simulink model "Parsim_for_3level"  (R2024b)
settings: Solver=FixedStepDiscrete  StartTime=0.0  StopTime=1  FixedStep=Ts  RelTol=1e-3
PreLoadFcn:
  | Net_improve_init;L=Lac_MV;Ts=20e-6;Tctrl=Ts;Rac_MV=1;
PostLoadFcn:
  | Net_improve_init;L=Lac_MV;Ts=20e-6;Tctrl=Ts;Rac_MV=1;
InitFcn:
  | Net_improve_init;L=Lac_MV;Ts=20e-6;Tctrl=Ts;Rac_MV=1;
undefined symbols (not defined in the file or in its folder): C1, dend, DiscIntNeverNeededParam, fs, Lac_MV, numd, Pref, R1, Vac_peak_MV, Vdc
libraries: spsIGBTDiodeLib x12, powerlib_extras x10, spsControlledVoltageSourceLib x8, spsCurrentMeasurementLib x6, spsSeriesRLCBranchLib x6, spsVoltageMeasurementLib x6, spsThreePhaseVIMeasurementLib x4, spsGroundLib x4, spsIdealSwitchLib x2, spsPower3phInstantaneousLib x2, simulink x2, spsThreePhaseSeriesRLCBranchLib x2
(part 1 of 2)
Description:
  | The Model initialization function Callback automatically
  | 
  | sets the sample time  to 2e-6 sec.  and loads the initial
  | 
  | states vector xInitial. The initial state vector is saved in the
  | 
  | power_acdrive_init.mat file.
  | 
  | 
  | 
  | Check  the Initial state checkbox in the Simulation
  | 
  | parameters/Workspace I/O to start in steady state with a
  | 
  | speed of 120 rad/s and a torque of 0 N.m/s,
  | 
  | 
  | Copyright 2008-2015 The MathWorks, Inc.
settings Model: Creator=WeiLi  LastModifiedBy=KeXing
settings SolverCC: AlgebraicLoopSolver=TrustRegion
settings DataIOCC: SaveFinalState=on  SaveFormat=Array  SignalLoggingSaveFormat=ModelDataLogs  SaveOutput=off  SaveTime=off  ReturnWorkspaceOutputs=off  SignalLoggingName=sigsOut
settings OptimizationCC: BlockReduction=off  ExpressionDepthLimit=2147483647  InitFltsAndDblsToZero=on  LifeSpan=inf
settings DebuggingCC: SaveWithParameterizedLinksMsg=none  UnderspecifiedInitializationDetection=Classic  MergeDetectMultiDrivingBlocksExec=none  CheckExecutionContextPreStartOutputMsg=on  SignalResolutionControl=TryResolveAllWithWarning  MultiTaskDSMMsg=warning  MultiTaskCondExecSysMsg=none  FcnCallInpInsideContextMsg=warning  UnconnectedInputMsg=warning  UnconnectedLineMsg=warning  StateNameClashWarn=warning  SFUnexpectedBacktrackingDiag=warning  SFNoUnconditionalDefaultTransitionDiag=warning  SFExecutionAtInitializationDiag=none  ArithmeticOperatorsInVariantConditions=warning
settings HardwareCC: ProdBitPerPointer=32  ProdBitPerSizeT=32  ProdBitPerPtrDiffT=32  ProdLargestAtomicFloat=None  ProdIntDivRoundTo=Undefined  ProdEndianess=Unspecified  ProdWordSize=32  ProdHWDeviceType=32-bit Generic  TargetUnknown=on
settings ModelReferenceCC: EnableRefExpFcnMdlSchedulingChecks=on  PropagateSignalLabelsOutOfModel=off
settings SFSimCC: SimUseLocalCustomCode=off  CustomCodeUndefinedFunction=UseInterfaceOnly
settings RTWCC: RTWUseLocalCustomCode=off  GPUComputeCapability=3.5
settings CodeAppCC: StateflowObjectComments=on
settings GRTTargetCC: TargetFcnLib=ansi_tfl_tmw.mat  TargetLangStandard=C89/C90 (ANSI)  CombineOutputUpdateFcns=off  GRTInterface=on
settings ConfigComp: CovMetricSettings=dw  CovSaveCumulativeToWorkspaceVar=on  CovSaveSingleToWorkspaceVar=on  CovExternalEMLEnable=off
settings SimscapeCC: SimscapeNormalizeSystem=off

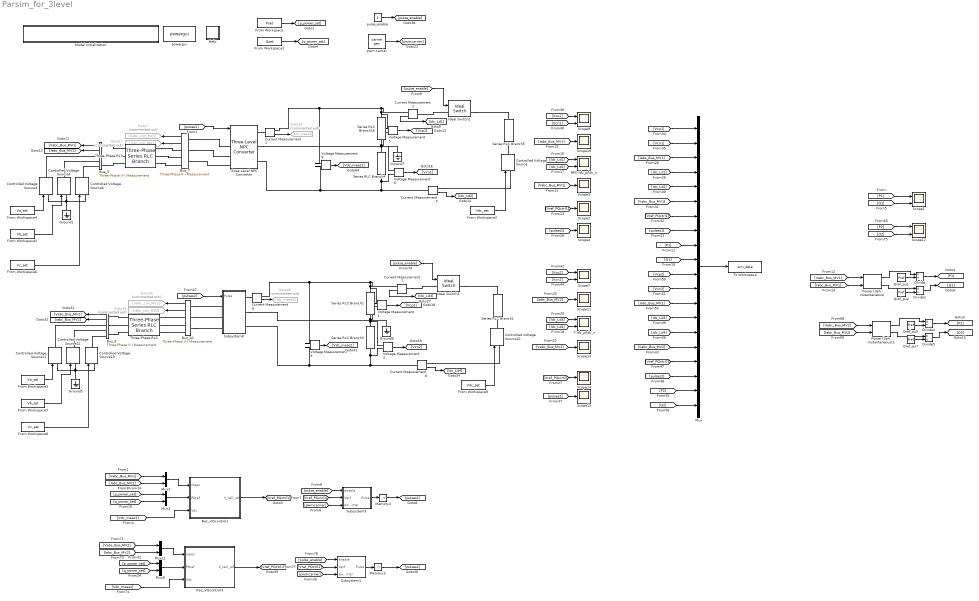
== system Parsim_for_3level ==
  Bus_{5,7,9..10} (4 alike) : spsThreePhaseVIMeasurementLib/Three-Phase V-I Measurement  VoltageMeasurement=phase-to-ground  SetLabelV=off  LabelV=Vabc  Vpu=off  VpuLL=off  CurrentMeasurement=yes  SetLabelI=off  LabelI=Iabc  Ipu=off  Pbase=P_AC  Vbase=V_AC_prim  OutputType=Complex  PhasorSimulation=off  PSBequivalent=0
  Controlled Voltage Source : spsControlledVoltageSourceLib/Controlled Voltage Source  Initialize=on  Source_Type=DC  Amplitude=3000  Phase=0  Frequency=0  Measurements=None
  Controlled Voltage Source10 : spsControlledVoltageSourceLib/Controlled Voltage Source  Initialize=on  Source_Type=DC  Amplitude=3000  Phase=0  Frequency=0  Measurements=None
  Controlled Voltage Source{3..4,6,11..13} (6 alike) : spsControlledVoltageSourceLib/Controlled Voltage Source  Initialize=off  Source_Type=AC  Amplitude=0  Phase=0  Frequency=fs  Measurements=None
  Current Measurement{1..2,5..8} (6 alike) : spsCurrentMeasurementLib/Current Measurement  PhasorSimulation=off  OutputType=Complex  PSBequivalent=0
  Divide{,1,4..5} (4 alike) : Product  Inputs=*/
  From Workspace : FromWorkspace  VariableName=Pset
  From Workspace1 : FromWorkspace  VariableName=Qset
  From Workspace2 : FromWorkspace  VariableName=Vdc_set  SampleTime=Ts
  From Workspace3 : FromWorkspace  VariableName=Va_set  SampleTime=Ts
  From Workspace4 : FromWorkspace  VariableName=Va_set  SampleTime=Ts
  From Workspace5 : FromWorkspace  VariableName=Vb_set  SampleTime=Ts
  From Workspace6 : FromWorkspace  VariableName=Vc_set  SampleTime=Ts
  From Workspace7 : FromWorkspace  VariableName=Vb_set  SampleTime=Ts
  From Workspace8 : FromWorkspace  VariableName=Vc_set  SampleTime=Ts
  From Workspace9 : FromWorkspace  VariableName=Vdc_set  SampleTime=Ts
  Goto10 : Goto  Commented=on  GotoTag=Idc_meas1
  Goto17 : Goto  Commented=on  GotoTag=iabc_con_MV1
  Goto28 : Goto  Commented=on  GotoTag=Idc_meas2
  Goto30 : Goto  Commented=on  GotoTag=Vabc_con_MV2
  Goto33 : Goto  Commented=on  GotoTag=iabc_con_MV2
  Goto7 : Goto  Commented=on  GotoTag=Vabc_con_MV1
  Ground{1,5..7} (4 alike) : spsGroundLib/Ground  LConnTagsString=a
  Help : Subsystem  mask(OpDoc){docfile=../Help/help.html}
      mask init:
      | %patch([1,1,0,0,.8,1],[.8,0,0,1,1,.8],[.8 .8 .8]);
      | %patch([.15 .78 .78 .15 .15],[.8 .8 .83 .83 .8],[.9 .9 .9]);
      | %patch([.15 .78 .78 .15 .15],[.7 .7 .73 .73 .8],[.9 .9 .9]);
      | %patch([.15 .78 .78 .15 .15],[.6 .6 .63 .63 .6],[.9 .9 .9]);
      | %patch([.15 .78 .78 .15 .15],[.5 .5 .53 .53 .5],[.9 .9 .9]);
      | %patch([.15 .78 .78 .15 .15],[.4 .4 .43 .43 .4],[.9 .9 .9]);
      settings: OpenFcn=OpHelp_cb(gcb);
      mask Display: image(imread('opdoc.bmp'))
  Ideal Switch2 : spsIdealSwitchLib/Ideal Switch  Ron=0.001  Lon=0  IC=0  Rs=1e9  Cs=inf  Measurements=on
  Ideal Switch3 : spsIdealSwitchLib/Ideal Switch  Ron=0.001  Lon=0  IC=0  Rs=1e9  Cs=inf  Measurements=on
  Memory2 : Memory
  Memory3 : Memory
  Model Initialization : Subsystem  mask(Model Functions){InitFcnX=Net_improve_init;L=Lac_MV;Ts=20e-6;Tctrl=Ts;Rac_MV=1;, prel=on, posl=on, inif=on, strf=off}
      mask prompts: InitFcnX "Initialisation"; prel "Preload Function"; posl "PostLoad Function"; inif "InitFcn"; strf "StartFcn"
      mask init:
      | currentBlock = gcb;
      | root = bdroot(currentBlock);
      | 
      | if ~strcmp(get_param(root,'BlockDiagramType'),'library')
      |     if prel==1
      |         set_param(root, 'PreLoadFcn', InitFcnX);
      |     else
      |         set_param(root, 'PreLoadFcn', '');
      |     end
      |     if inif==1
      |         set_param(root, 'InitFcn', InitFcnX);
      |     else
      |         set_param(root, 'InitFcn', '');
      |     end
      |     if strf==1
      |         set_param(root, 'StartFcn', InitFcnX);
      |     else
      |         set_param(root, 'StartFcn', '');
      |     end
      |     if posl==1
      |         set_param(root, 'PostLoadFcn', InitFcnX);
      |     else
      |         set_param(root, 'PostLoadFcn', '');
      |     end
      | end
      | 
      | pos = get_param(currentBlock, 'Position');
      | width = pos(3) - pos(1); height = pos(4) - pos(2);
      | txt = [ upper(root) '\n' '- InitFcn. . . . . '  get_param(root, 'InitFcn') ];
      settings: CopyFcn=set_param(gcb,'LinkStatus','none')
      mask Display: text(5, height*0.5, txt, 'horizontalAlignment', 'left', 'verticalAlignment', 'middle') ;
  Mux : Mux  Inputs=20
  Mux{1..2,8,11} (4 alike) : Mux  Inputs=2
  NPC-Idc_p/Idc_n : Scope  NumInputPorts=2
  "Power (3ph, Instantaneous)" : spsPower3phInstantaneousLib/Power (3ph, Instantaneous)
  "Power (3ph, Instantaneous)2" : spsPower3phInstantaneousLib/Power (3ph, Instantaneous)
  Qref_pu{1..2,5,7} (4 alike) : Constant  Value=Pref
  Rec_VQcontrol1 : Subsystem  mask(converter controller){cm=off, base=[Pref, Vac_peak_MV*sqrt(3/2), Vdc/2, fs], LRx=[Lac_MV, Rac_MV], LRx_inpu=off, Kd=[0.3  2]*10/6  %was [1 0.1]   ; [0.1  1]*1, Kp=[0.3 1]*1     %was [1 0.1]   ; [0.1  1]*1, Kvdc=[2 10]*1;   %was [0.5 1]*20 for Cdc=320uF, Vabc_lim=[-1 1], limitVdq=1.1, nadv=6, xtrIctrl1=[0.4 10 10 -10], Ts=Tctrl}
      mask prompts: cm "control mode (check VQ/uncheck PQ), only one terminal in VQ mode"; base "base value for power(VA), ac voltage(V), dc voltage to ground(V), and frequenvy(Hz) [Sb, Vb, Vdcb,freq]"; LRx "commutation inductance and resistance [Lx, Rx]"; LRx_inpu "[Lx, Rx] in pu if checked/ SI unchecked"; Kd "Kp Ki for d-axis PI control [kp ki]"; Kp "Kp Ki for q-axis PI control [kp ki]"; Kvdc "Kp Ki for Vdc PI control [kp ki]"; Vabc_lim "output Vabc limit [min max]"; limitVdq "limit for Vd,Vq (pu, default = 1.1)"; nadv "nb of time step to compesate for delay (default=1)"; xtrIctrl1 "[kp, kp, limitmax, limitmin] for current control (default=[0.4, 10, 10, -10])"
      mask help:
      | input 1, 6 dimentions, Vabc, Iabc, (SI)
      | input 2, 2 dimentions, Pref, Qref (PU)
      | input 3, 6 dimentions, Vcap at up arm a, lower arm a, up arm b, lower arm b, up arm c and lower arm c.
      | input 4, 1 dimention, pulse on
      | input 5, 1 dimention
      |
      | power or current directions: to go into grid is positive
      mask init:
      | if cm==0;
      |     x=['PQ\nmode'];
      | else
      |     x=['VQ\nmode'];
      | end
      | 
      | Sb=base(1);            %VA 3phase power base;
      | Vb=base(2);       %V, line-line rms voltage base
      | Ib=Sb/(sqrt(3)*Vb); %A, rms current base
      | Zb=Vb^2/Sb ;        %ohm, impedence base
      | Vdc=base(3);      %V Vdc+ to ground or ground to Vdc- 
      | frq=base(4);
      | 
      | if LRx_inpu
      |     Rxpu=LRx(2);
      |     Lxpu=LRx(1);
      | else
      |     Rxpu=LRx(2)/Zb;
      |     Lxpu=LRx(1)*2*pi*frq/Zb;
      | end;
      | 
      | ks=Vdc*sqrt(3/2)/Vb;     % ma=1/ks for 1pu dc ->1pu ac;
      | 
      | Kp=Kd;
      mask DialogControl ParameterTabVar0 Prompt: parameters
      mask DialogControl ParameterTabVar01 Prompt: advanced
      mask Display: disp (x);
  Rec_VQcontrol3 : Subsystem  mask(converter controller){cm=off, base=[Pref, Vac_peak_MV*sqrt(3/2), Vdc/2, fs], LRx=[Lac_MV, Rac_MV], LRx_inpu=off, Kd=[0.3  2]*10/6  %was [1 0.1]   ; [0.1  1]*1, Kp=[0.3 1]*1     %was [1 0.1]   ; [0.1  1]*1, Kvdc=[2 10]*1;   %was [0.5 1]*20 for Cdc=320uF, Vabc_lim=[-1 1], limitVdq=1.1, nadv=6, xtrIctrl1=[0.4 10 10 -10], Ts=Tctrl}
      mask prompts: cm "control mode (check VQ/uncheck PQ), only one terminal in VQ mode"; base "base value for power(VA), ac voltage(V), dc voltage to ground(V), and frequenvy(Hz) [Sb, Vb, Vdcb,freq]"; LRx "commutation inductance and resistance [Lx, Rx]"; LRx_inpu "[Lx, Rx] in pu if checked/ SI unchecked"; Kd "Kp Ki for d-axis PI control [kp ki]"; Kp "Kp Ki for q-axis PI control [kp ki]"; Kvdc "Kp Ki for Vdc PI control [kp ki]"; Vabc_lim "output Vabc limit [min max]"; limitVdq "limit for Vd,Vq (pu, default = 1.1)"; nadv "nb of time step to compesate for delay (default=1)"; xtrIctrl1 "[kp, kp, limitmax, limitmin] for current control (default=[0.4, 10, 10, -10])"
      mask help:
      | input 1, 6 dimentions, Vabc, Iabc, (SI)
      | input 2, 2 dimentions, Pref, Qref (PU)
      | input 3, 6 dimentions, Vcap at up arm a, lower arm a, up arm b, lower arm b, up arm c and lower arm c.
      | input 4, 1 dimention, pulse on
      | input 5, 1 dimention
      |
      | power or current directions: to go into grid is positive
      mask init: same as Parsim_for_3level/Rec_VQcontrol1
      mask DialogControl ParameterTabVar0 Prompt: parameters
      mask DialogControl ParameterTabVar01 Prompt: advanced
      mask Display: disp (x);
  Scope{1,7,9,12} (4 alike) : Scope  NumInputPorts=2
  Scope{2..4,10..11,13..15} (8 alike) : Scope
  Series RLC Branch1 : spsSeriesRLCBranchLib/Series RLC Branch  LConnTagsString=__new0  RConnTagsString=__new0  BranchType=R  Resistance=3e3^2/(Pref)/10*2  Inductance=1e-3  SetiL0=off  InitialCurrent=0  Capacitance=C1  Setx0=off  InitialVoltage=0  Measurements=None
  Series RLC Branch{2..4,16} (4 alike) : spsSeriesRLCBranchLib/Series RLC Branch  LConnTagsString=__new0  RConnTagsString=__new0  BranchType=C  Resistance=R1  Inductance=1e-3  SetiL0=off  InitialCurrent=0  Capacitance=C1  Setx0=off  InitialVoltage=0  Measurements=None
  Series RLC Branch5 : spsSeriesRLCBranchLib/Series RLC Branch  LConnTagsString=__new0  RConnTagsString=__new0  BranchType=R  Resistance=3e3^2/(Pref)/10*2  Inductance=1e-3  SetiL0=off  InitialCurrent=0  Capacitance=C1  Setx0=off  InitialVoltage=0  Measurements=None
  Subsystem1 : Subsystem
  Subsystem8 : Subsystem
  Subsystem9 : Subsystem
  T-Idc_p/Idc_n : Scope  NumInputPorts=2
  Three-Level NPC Converter : spsThreeLevelNPCConverterLib/Three-Level NPC Converter  ModelType=Switching devices  Ron=IGBT_Ron  Rs=1e5  Cs=IGBT_Cs  Vforward=[0,0]  Ron_Diode=1e-3  Rs_Diode=1e6  Cs_Diode=inf  Vf_Diode=1e-3  Rs_CurrentSource=inf  Ron_ACsource=1e-3
      settings: LibrarySourceBlock=|
      | sps_lib/Power Electronics/Three-Level
      | NPC Converter
  Three-Phase RL3 : spsThreePhaseSeriesRLCBranchLib/Three-Phase Series RLC Branch  LConnTagsString=A|B|C  RConnTagsString=A|B|C  BranchType=RL  Resistance=Rac_MV  Inductance=Lac_MV  Capacitance=1e-6  Measurements=None
  Three-Phase RL5 : spsThreePhaseSeriesRLCBranchLib/Three-Phase Series RLC Branch  LConnTagsString=A|B|C  RConnTagsString=A|B|C  BranchType=RL  Resistance=Rac_MV  Inductance=Lac_MV  Capacitance=1e-6  Measurements=None
  To Workspace : ToWorkspace  VariableName=sim_data  SampleTime=-1
      settings: Save2DSignal=2-D array (concatenate along first dimension)
  Voltage Measurement{1..3,5..6,8} (6 alike) : spsVoltageMeasurementLib/Voltage Measurement  PhasorSimulation=off  OutputType=Complex  PSBequivalent=0
  powergui : spspowerguiLib/powergui  Priority=2  SimulationMode=Discrete  SampleTime=Ts  frequency=60  Iterations=50  frequencyindice=0  Pbase=100e6  ErrMax=1e-4  UnitsV=kV  UnitsW=MW  buscounter=0  FunctionMessages=off  echomessages=off  EnableUseOfTLC=off  CurrentSourceSwitches=off  DisableSnubberDevices=off  DisableRonSwitches=off  DisableVfSwitches=off  DisplayEquations=off  AutomaticDiscreteSolvers=off  SolverType=Backward Euler  Interpol=off  ExternalGateDelay=off  methode=off  Ts=0  x0status=blocks  SPID=off  SwTol=0  HookPort=off  NonlinearTolerance=1e-4  nMaxIteration=100  ContinueOnMaxIteration=off  RestoreLinks=warning  ResistiveCurrentMeasurement=off  Frange=[0:2:500]  Ylog=off  Xlog=on  ShowGrid=off  save=off  variable=ZData  structure=VI  ZoomFFT=off  StartTime=9  cycles=10  DisplayStyle=2  fundamental=300/pi  FreqAxis=off  MaxFrequency=1000  frequencyindicesteady=1  RmsSteady=1  display=off
  pulse_enable : Constant
  pwm carrier : libMMCcpuv2/carrier gen  fc=f_cari  range=[1 0]  Ms=3  Ns=1
  wires:
  pwm carrier/1 -> [pwmcarrier]
  From Workspace1/1 -> [q_power_set]
  pulse_enable/1 -> [pulse_enable]
  From Workspace/1 -> [p_power_set]
  Current Measurement1/1 -> Goto10/1
  From Workspace2/1 -> Controlled Voltage Source/1
  Bus_5/1 -> [Vabc_Bus_MV1]
  [pulses1] -> Three-Level NPC Converter/1
  Bus_7/1 -> Goto7/1
  Bus_7/2 -> Goto17/1
  [Iabc_Bus_MV1] -> "Power (3ph, Instantaneous)"/2
  [p_power_set] -> Mux1/1
  [Q1] -> Scope1/2
  Mux1/1 -> Rec_VQcontrol1/2(PQref)
  Qref_pu2/1 -> Divide1/2
  Qref_pu1/1 -> Divide/2
  [P1] -> Scope1/1
  [Vdc_meas1] -> Rec_VQcontrol1/3(Vdc)
  Divide1/1 -> [Q1]
  Rec_VQcontrol1/1(V_cell_ref) -> [Vref_PQctrl1]
  [pulse_enable] -> Ideal Switch2/1
  Current Measurement5/1 -> [Idc_Ld2]
  Voltage Measurement6/1 -> [Vcn1]
  Subsystem9/1(Pulse) -> Memory2/1
  [pwmcarrier] -> Subsystem9/3(pwmcarrier)
  Mux2/1 -> Rec_VQcontrol1/1(meas)
  [Vref_PQctrl1] -> Subsystem9/2(Verf)
  [pulse_enable] -> Subsystem9/1(enable)
  Current Measurement2/1 -> [Idc_Ld1]
  [Iabc_Bus_MV1] -> Mux2/2
  Bus_5/2 -> [Iabc_Bus_MV1]
  Voltage Measurement8/1 -> [Vdc_meas1]
  Voltage Measurement5/1 -> [Vcp1]
  From Workspace6/1 -> Controlled Voltage Source6/1
  From Workspace5/1 -> Controlled Voltage Source4/1
  [Vabc_Bus_MV1] -> Mux2/1
  Divide/1 -> [P1]
  Memory2/1 -> [pulses1]
  [Vabc_Bus_MV1] -> "Power (3ph, Instantaneous)"/1
  From Workspace4/1 -> Controlled Voltage Source3/1
  "Power (3ph, Instantaneous)"/1 -> Divide/1
  [q_power_set] -> Mux1/2
  "Power (3ph, Instantaneous)"/2 -> Divide1/1
  [pulse_enable] -> Ideal Switch3/1
  Voltage Measurement3/1 -> [Vdc_meas2]
  From Workspace7/1 -> Controlled Voltage Source12/1
  From Workspace3/1 -> Controlled Voltage Source11/1
  [pwmcarrier] -> Subsystem1/3(pwmcarrier)
  [Vref_PQctrl2] -> Subsystem1/2(Verf)
  Subsystem1/1(Pulse) -> Memory3/1
  [pulse_enable] -> Subsystem1/1(enable)
  Qref_pu5/1 -> Divide4/2
  Memory3/1 -> [pulses2]
  [Iabc_Bus_MV2] -> "Power (3ph, Instantaneous)2"/2
  [Vdc_meas2] -> Rec_VQcontrol3/3(Vdc)
  From Workspace8/1 -> Controlled Voltage Source13/1
  [P2] -> Scope12/1
  Divide5/1 -> [Q2]
  Divide4/1 -> [P2]
  [Q2] -> Scope12/2
  Mux8/1 -> Rec_VQcontrol3/2(PQref)
  "Power (3ph, Instantaneous)2"/1 -> Divide4/1
  Mux11/1 -> Rec_VQcontrol3/1(meas)
  From Workspace9/1 -> Controlled Voltage Source10/1
  Bus_10/2 -> Goto33/1
  Voltage Measurement2/1 -> [Vcn2]
  "Power (3ph, Instantaneous)2"/2 -> Divide5/1
  Bus_9/1 -> [Vabc_Bus_MV2]
  [Vabc_Bus_MV2] -> "Power (3ph, Instantaneous)2"/1
  Current Measurement8/1 -> [Idc_Ld4]
  [Iabc_Bus_MV2] -> Mux11/2
  Current Measurement6/1 -> Goto28/1
  Bus_10/1 -> Goto30/1
  [pulses2] -> Subsystem8/1(Pulse)
  Bus_9/2 -> [Iabc_Bus_MV2]
  [Vabc_Bus_MV2] -> Mux11/1
  Rec_VQcontrol3/1(V_cell_ref) -> [Vref_PQctrl2]
  Current Measurement7/1 -> [Idc_Ld3]
  [q_power_set] -> Mux8/2
  Qref_pu7/1 -> Divide5/2
  Voltage Measurement1/1 -> [Vcp2]
  [Vref_PQctrl1] -> Scope2/1
  [Q1] -> Mux/10
  [Vref_PQctrl1] -> Mux/7
  [Vcp1] -> Mux/1
  [Iabc_Bus_MV1] -> Mux/3
  [Iabc_Bus_MV2] -> Mux/13
  [Vabc_Bus_MV2] -> Mux/16
  Mux/1 -> To Workspace/1
  [Vabc_Bus_MV2] -> Scope13/1
  [Vcn2] -> Scope7/2
  [Vabc_Bus_MV1] -> Mux/6
  [pulses2] -> Mux/18
  [Q2] -> Mux/20
  [Vcp1] -> Scope9/1
  [P1] -> Mux/9
  [Idc_Ld3] -> T-Idc_p/Idc_n/1
  [Vcp2] -> Mux/11
  [Idc_Ld3] -> Mux/14
  [Idc_Ld2] -> NPC-Idc_p/Idc_n/2
  [Idc_Ld4] -> Mux/15
  [Iabc_Bus_MV2] -> Scope11/1
  [Idc_Ld4] -> T-Idc_p/Idc_n/2
  [Iabc_Bus_MV1] -> Scope10/1
  [Vref_PQctrl2] -> Scope14/1
  [Idc_Ld2] -> Mux/5
  [pulses1] -> Scope4/1
  [Vcp2] -> Scope7/1
  [Vabc_Bus_MV1] -> Scope3/1
  [pulses1] -> Mux/8
  [pulses2] -> Scope15/1
  [Vref_PQctrl2] -> Mux/17
  [Vcn1] -> Scope9/2
  [Vcn1] -> Mux/2
  [P2] -> Mux/19
  [Idc_Ld1] -> NPC-Idc_p/Idc_n/1
  [Vcn2] -> Mux/12
  [Idc_Ld1] -> Mux/4
  [p_power_set] -> Mux8/1
  connections:
  Current Measurement1/RConn1 -- Voltage Measurement8/LConn1 -- Voltage Measurement5/LConn1 -- Series RLC Branch16/LConn1 -- Current Measurement2/RConn1
  Voltage Measurement8/LConn2 -- Three-Level NPC Converter/RConn3 -- Current Measurement5/LConn1 -- Series RLC Branch4/RConn1 -- Voltage Measurement6/LConn2
  Series RLC Branch16/RConn1 -- Voltage Measurement5/LConn2 -- Three-Level NPC Converter/RConn2 -- Series RLC Branch4/LConn1 -- Voltage Measurement6/LConn1 -- Ground7/LConn1
  Ground1/LConn1 -- Controlled Voltage Source6/LConn1 -- Controlled Voltage Source3/LConn1 -- Controlled Voltage Source4/LConn1
  Three-Phase RL3/RConn1 -- Bus_7/RConn1
  Bus_5/LConn2 -- Three-Phase RL3/LConn2
  Three-Level NPC Converter/LConn3 -- Bus_7/LConn3
  Bus_7/LConn2 -- Three-Level NPC Converter/LConn2
  Bus_5/LConn3 -- Three-Phase RL3/LConn3
  Bus_5/RConn1 -- Controlled Voltage Source3/RConn1
  Bus_5/RConn3 -- Controlled Voltage Source6/RConn1
  Three-Phase RL3/RConn2 -- Bus_7/RConn2
  Bus_7/LConn1 -- Three-Level NPC Converter/LConn1
  Bus_5/LConn1 -- Three-Phase RL3/LConn1
  Bus_5/RConn2 -- Controlled Voltage Source4/RConn1
  Current Measurement2/LConn1 -- Ideal Switch2/LConn1
  Three-Level NPC Converter/RConn1 -- Current Measurement1/LConn1
  Ideal Switch2/RConn1 -- Series RLC Branch5/RConn1
  Three-Phase RL3/RConn3 -- Bus_7/RConn3
  Current Measurement5/RConn1 -- Controlled Voltage Source/LConn1
  Series RLC Branch5/LConn1 -- Controlled Voltage Source/RConn1
  Controlled Voltage Source11/LConn1 -- Controlled Voltage Source12/LConn1 -- Ground5/LConn1 -- Controlled Voltage Source13/LConn1
  Voltage Measurement2/LConn1 -- Series RLC Branch3/LConn1 -- Subsystem8/RConn2 -- Ground6/LConn1 -- Series RLC Branch2/RConn1 -- Voltage Measurement1/LConn2
  Current Measurement6/RConn1 -- Voltage Measurement3/LConn1 -- Series RLC Branch2/LConn1 -- Voltage Measurement1/LConn1 -- Current Measurement7/RConn1
  Voltage Measurement3/LConn2 -- Subsystem8/RConn3 -- Current Measurement8/LConn1 -- Series RLC Branch3/RConn1 -- Voltage Measurement2/LConn2
  Three-Phase RL5/LConn1 -- Bus_9/LConn1
  Bus_10/LConn1 -- Subsystem8/LConn1
  Three-Phase RL5/RConn2 -- Bus_10/RConn2
  Bus_9/LConn3 -- Three-Phase RL5/LConn3
  Current Measurement7/LConn1 -- Ideal Switch3/LConn1
  Three-Phase RL5/RConn3 -- Bus_10/RConn3
  Bus_10/LConn2 -- Subsystem8/LConn2
  Bus_10/LConn3 -- Subsystem8/LConn3
  Bus_9/RConn1 -- Controlled Voltage Source11/RConn1
  Bus_9/LConn2 -- Three-Phase RL5/LConn2
  Bus_9/RConn2 -- Controlled Voltage Source12/RConn1
  Three-Phase RL5/RConn1 -- Bus_10/RConn1
  Controlled Voltage Source10/RConn1 -- Series RLC Branch1/LConn1
  Ideal Switch3/RConn1 -- Series RLC Branch1/RConn1
  Subsystem8/RConn1 -- Current Measurement6/LConn1
  Bus_9/RConn3 -- Controlled Voltage Source13/RConn1
  Current Measurement8/RConn1 -- Controlled Voltage Source10/LConn1

== system Parsim_for_3level/Help ==

== system Parsim_for_3level/Model Initialization ==

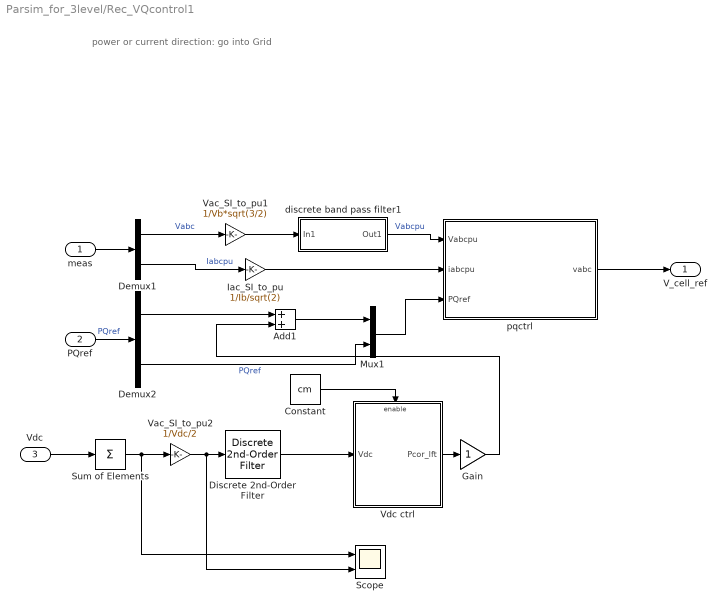
== system Parsim_for_3level/Rec_VQcontrol1 ==
  note: power or current direction: go into Grid
  meas : Inport
  PQref : Inport  Port=2
  Vdc : Inport  Port=3
  Add1 : Sum
  Constant : Constant  Value=cm
  Demux1 : Demux  Outputs=[3 3 ]
  Demux2 : Demux  Outputs=2
  Discrete 2nd-Order Filter : powerlib_extras/Discrete  Control Blocks/Discrete  2nd-Order Filter  FilterType=Lowpass  Fo=90  Zeta=0.707  Ts=Ts  Initialize=off  Vac_Init=[0.8 -25 60]  Vdc_Init=-0.4  PlotResponse=off  param1=[1 500 1]
  Gain : Gain
  Iac_SI_to_pu : Gain  Gain=1/Ib/sqrt(2)
  Mux1 : Mux  Inputs=2
  Scope : Scope  NumInputPorts=2
  Sum of Elements : Sum  Inputs=+
  Vac_SI_to_pu1 : Gain  Gain=1/Vb*sqrt(3/2)
  Vac_SI_to_pu2 : Gain  Gain=1/Vdc/2  SampleTime=Ts
  Vdc ctrl : Subsystem
  discrete band pass filter1 : Subsystem  mask(discrete transfer Fcn generator){Fo=frq, adj1=1, inistate=0, Ts=Ts, bodedw=off}
      mask prompts: Fo "F0 (Hz)"; adj1 "adj (1 for no adjustment, larger adj for wider band pass)"; inistate "Initial states"; Ts "Sample time (must be explicite)"; bodedw "draw Bode diagram of filter"
      mask help:
      | This block transfer a continous TF to a discrete TF
      | using Bilinear (Tustin) approximation
      mask init:
      | AD1=tf([1 0],1);
      | 
      | %second order
      | % Fo=50; %cut off freq.
      | % omega0=Fo*2*pi;
      | % adj1=3;   %adjustment 1
      | Zeta= 0.707*adj1; %Damping factor Zeta ( Q = 1 / (2*Zeta) ):
      | Wo=2*pi*Fo;
      | % str=sprintf(' Fo=%iHz\n\n',Fo);
      |  n2=0; n1=0;n0=Wo*Wo;
      |  d2=1;d1=2*Zeta*Wo;d0=Wo*Wo;
      | numc=[n2 n1 n0];
      | denc=[d2 d1 d0];
      | AD3=tf(numc,denc);
      | 
      | AD4=AD1*AD3;
      | [mag1,pha1]=bode(AD4,Wo);
      | mag0=mag1;
      | AD=AD4/mag0;
      | 
      | if bodedw==1
      |     figure;
      |     h=bodeplot(AD1,AD3,AD);
      |     setoptions(h,'FreqUnits','Hz');
      |     grid on;
      |     title(['Bode Diagram, adj=',num2str(adj1)]);
      | end;
      |     
      | % gg=tf(num,den);
      | ggd=c2d(AD,Ts,'tustin');
      | [numd,dend] = tfdata(ggd,'v');
  pqctrl : Subsystem
  V_cell_ref : Outport  VectorParamsAs1DForOutWhenUnconnected=off
  wires:
  Constant/1 -> Vdc ctrl/Enable
  Vac_SI_to_pu1/1 -> discrete band pass filter1/1(In1)
  Vac_SI_to_pu2/1 -> Scope/2, Discrete 2nd-Order Filter/1
  Vdc/1 -> Sum of Elements/1
  Discrete 2nd-Order Filter/1 -> Vdc ctrl/1(Vdc)
  Mux1/1 -> pqctrl/3(PQref)
  Demux2/2 -> Mux1/2  "PQref"
  Add1/1 -> Mux1/1
  Vdc ctrl/1(Pcor_lft) -> Gain/1
  Demux2/1 -> Add1/1
  Iac_SI_to_pu/1 -> pqctrl/2(iabcpu)
  Demux1/1 -> Vac_SI_to_pu1/1  "Vabc"
  Demux1/2 -> Iac_SI_to_pu/1  "Iabcpu"
  meas/1 -> Demux1/1
  discrete band pass filter1/1(Out1) -> pqctrl/1(Vabcpu)  "Vabcpu"
  PQref/1 -> Demux2/1  "PQref"
  pqctrl/1(vabc) -> V_cell_ref/1
  Sum of Elements/1 -> Scope/1, Vac_SI_to_pu2/1
  Gain/1 -> Add1/2

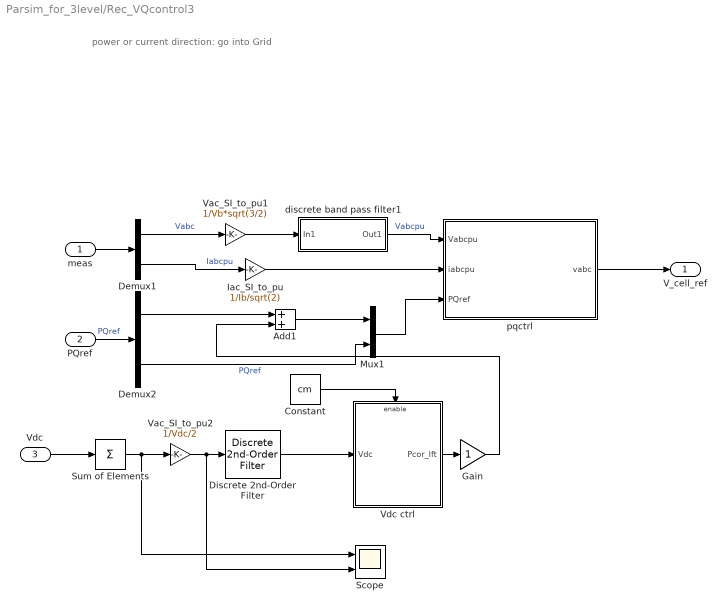
== system Parsim_for_3level/Rec_VQcontrol3 ==
  note: power or current direction: go into Grid
  meas : Inport
  PQref : Inport  Port=2
  Vdc : Inport  Port=3
  Add1 : Sum
  Constant : Constant  Value=cm
  Demux1 : Demux  Outputs=[3 3 ]
  Demux2 : Demux  Outputs=2
  Discrete 2nd-Order Filter : powerlib_extras/Discrete  Control Blocks/Discrete  2nd-Order Filter  FilterType=Lowpass  Fo=90  Zeta=0.707  Ts=Ts  Initialize=off  Vac_Init=[0.8 -25 60]  Vdc_Init=-0.4  PlotResponse=off  param1=[1 500 1]
  Gain : Gain
  Iac_SI_to_pu : Gain  Gain=1/Ib/sqrt(2)
  Mux1 : Mux  Inputs=2
  Scope : Scope  NumInputPorts=2
  Sum of Elements : Sum  Inputs=+
  Vac_SI_to_pu1 : Gain  Gain=1/Vb*sqrt(3/2)
  Vac_SI_to_pu2 : Gain  Gain=1/Vdc/2  SampleTime=Ts
  Vdc ctrl : Subsystem
  discrete band pass filter1 : Subsystem  mask(discrete transfer Fcn generator){Fo=frq, adj1=1, inistate=0, Ts=Ts, bodedw=off}
      mask prompts: Fo "F0 (Hz)"; adj1 "adj (1 for no adjustment, larger adj for wider band pass)"; inistate "Initial states"; Ts "Sample time (must be explicite)"; bodedw "draw Bode diagram of filter"
      mask help:
      | This block transfer a continous TF to a discrete TF
      | using Bilinear (Tustin) approximation
      mask init: same as Parsim_for_3level/Rec_VQcontrol1/discrete band pass filter1
  pqctrl : Subsystem
  V_cell_ref : Outport  VectorParamsAs1DForOutWhenUnconnected=off
  wires:
  Constant/1 -> Vdc ctrl/Enable
  Vac_SI_to_pu1/1 -> discrete band pass filter1/1(In1)
  Vac_SI_to_pu2/1 -> Scope/2, Discrete 2nd-Order Filter/1
  Vdc/1 -> Sum of Elements/1
  Discrete 2nd-Order Filter/1 -> Vdc ctrl/1(Vdc)
  Mux1/1 -> pqctrl/3(PQref)
  Demux2/2 -> Mux1/2  "PQref"
  Add1/1 -> Mux1/1
  Vdc ctrl/1(Pcor_lft) -> Gain/1
  Demux2/1 -> Add1/1
  Iac_SI_to_pu/1 -> pqctrl/2(iabcpu)
  Demux1/1 -> Vac_SI_to_pu1/1  "Vabc"
  Demux1/2 -> Iac_SI_to_pu/1  "Iabcpu"
  meas/1 -> Demux1/1
  discrete band pass filter1/1(Out1) -> pqctrl/1(Vabcpu)  "Vabcpu"
  PQref/1 -> Demux2/1  "PQref"
  pqctrl/1(vabc) -> V_cell_ref/1
  Sum of Elements/1 -> Scope/1, Vac_SI_to_pu2/1
  Gain/1 -> Add1/2

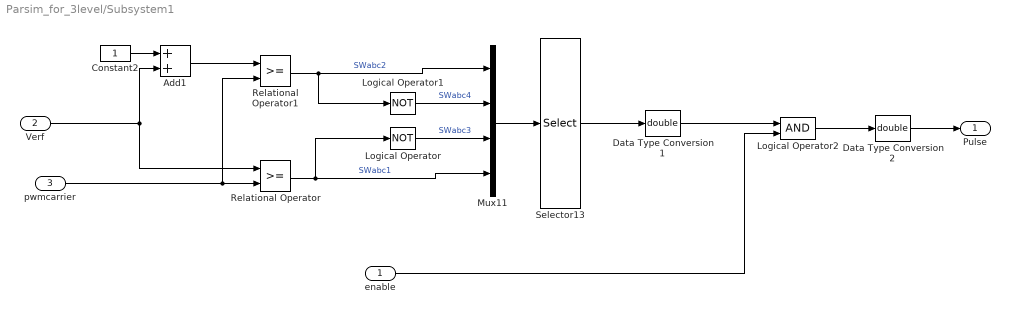
== system Parsim_for_3level/Subsystem1 ==
  enable : Inport
  Verf : Inport  Port=2
  pwmcarrier : Inport  Port=3
  Add1 : Sum
  Constant2 : Constant
  Data Type Conversion1 : DataTypeConversion  OutDataTypeStr=double  SaturateOnIntegerOverflow=off  RndMeth=Floor
  Data Type Conversion2 : DataTypeConversion  OutDataTypeStr=double  SaturateOnIntegerOverflow=off  RndMeth=Floor
  Logical Operator : Logic  Operator=NOT  AllPortsSameDT=off  OutDataTypeStr=boolean
  Logical Operator1 : Logic  Operator=NOT  AllPortsSameDT=off  OutDataTypeStr=boolean
  Logical Operator2 : Logic  AllPortsSameDT=off
  Mux11 : Mux
  Relational Operator : RelationalOperator  OutDataTypeStr=boolean  RndMeth=Simplest  InputSameDT=off
  Relational Operator1 : RelationalOperator  OutDataTypeStr=boolean  RndMeth=Simplest  InputSameDT=off
  Selector13 : Selector  InputPortWidth=12  IndexOptions=Index vector (dialog)  Indices=[10 1 7 4 11 2 8 5 12 3 9 6]  OutputSizes=1
  Pulse : Outport  VectorParamsAs1DForOutWhenUnconnected=off
  wires:
  pwmcarrier/1 -> Relational Operator/2, Relational Operator1/2
  Relational Operator1/1 -> Mux11/1, Logical Operator1/1  "SWabc2"
  Logical Operator/1 -> Mux11/3  "SWabc3"
  Relational Operator/1 -> Logical Operator/1, Mux11/4  "SWabc1"
  Constant2/1 -> Add1/1
  Add1/1 -> Relational Operator1/1
  Verf/1 -> Add1/2, Relational Operator/1
  Selector13/1 -> Data Type Conversion1/1
  Mux11/1 -> Selector13/1
  Logical Operator1/1 -> Mux11/2  "SWabc4"
  Data Type Conversion1/1 -> Logical Operator2/1
  enable/1 -> Logical Operator2/2
  Logical Operator2/1 -> Data Type Conversion2/1
  Data Type Conversion2/1 -> Pulse/1

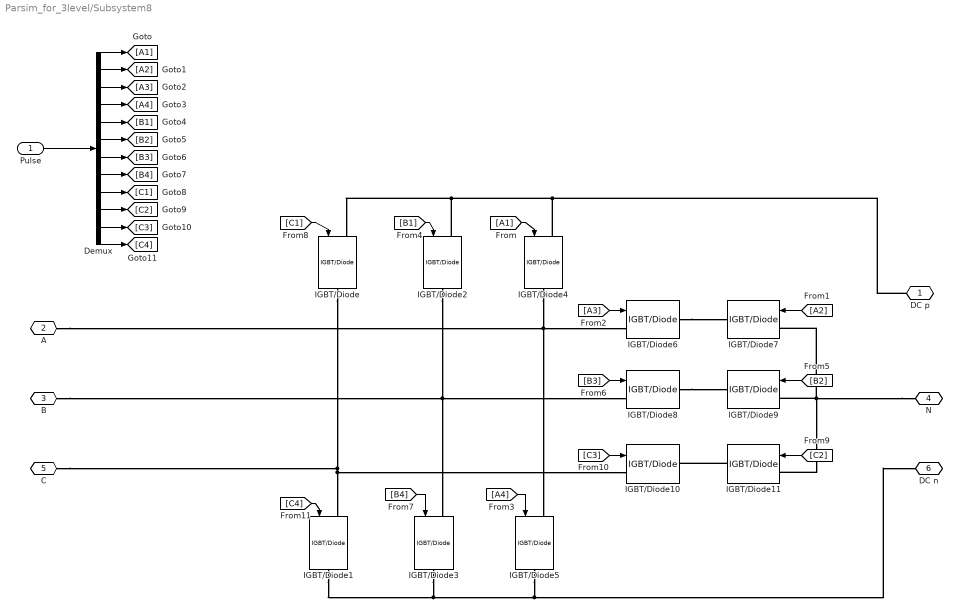
== system Parsim_for_3level/Subsystem8 ==
  Pulse : Inport
  Demux : Demux  Outputs=12
  IGBT/Diode{,1..11} (12 alike) : spsIGBTDiodeLib/IGBT//Diode  Ron=IGBT_Ron  Rs=IGBT_Rs  Cs=IGBT_Cs  Measurements=off
  DC p : PMIOPort  Side=Right
  A : PMIOPort  Port=2  Side=Left
  B : PMIOPort  Port=3  Side=Left
  N : PMIOPort  Port=4  Side=Right
  C : PMIOPort  Port=5  Side=Left
  DC n : PMIOPort  Port=6  Side=Right
  wires:
  [B1] -> IGBT/Diode2/1
  [C1] -> IGBT/Diode/1
  Pulse/1 -> Demux/1
  [C4] -> IGBT/Diode1/1
  [B4] -> IGBT/Diode3/1
  [A4] -> IGBT/Diode5/1
  [A2] -> IGBT/Diode7/1
  [A1] -> IGBT/Diode4/1
  Demux/1 -> [A1]
  Demux/12 -> [C4]
  Demux/2 -> [A2]
  Demux/3 -> [A3]
  Demux/4 -> [A4]
  Demux/5 -> [B1]
  Demux/6 -> [B2]
  Demux/7 -> [B3]
  Demux/8 -> [B4]
  Demux/9 -> [C1]
  Demux/10 -> [C2]
  Demux/11 -> [C3]
  [B2] -> IGBT/Diode9/1
  [C2] -> IGBT/Diode11/1
  [A3] -> IGBT/Diode6/1
  [B3] -> IGBT/Diode8/1
  [C3] -> IGBT/Diode10/1
  connections:
  IGBT/Diode4/RConn1 -- IGBT/Diode6/LConn1 -- IGBT/Diode5/LConn1 -- A/RConn1
  DC p/RConn1 -- IGBT/Diode4/LConn1 -- IGBT/Diode2/LConn1 -- IGBT/Diode/LConn1
  IGBT/Diode6/RConn1 -- IGBT/Diode7/RConn1
  IGBT/Diode2/RConn1 -- IGBT/Diode8/LConn1 -- B/RConn1 -- IGBT/Diode3/LConn1
  IGBT/Diode1/RConn1 -- IGBT/Diode3/RConn1 -- DC n/RConn1 -- IGBT/Diode5/RConn1
  IGBT/Diode8/RConn1 -- IGBT/Diode9/RConn1
  IGBT/Diode11/RConn1 -- IGBT/Diode10/RConn1
  IGBT/Diode/RConn1 -- IGBT/Diode10/LConn1 -- IGBT/Diode1/LConn1 -- C/RConn1
  N/RConn1 -- IGBT/Diode7/LConn1 -- IGBT/Diode11/LConn1 -- IGBT/Diode9/LConn1

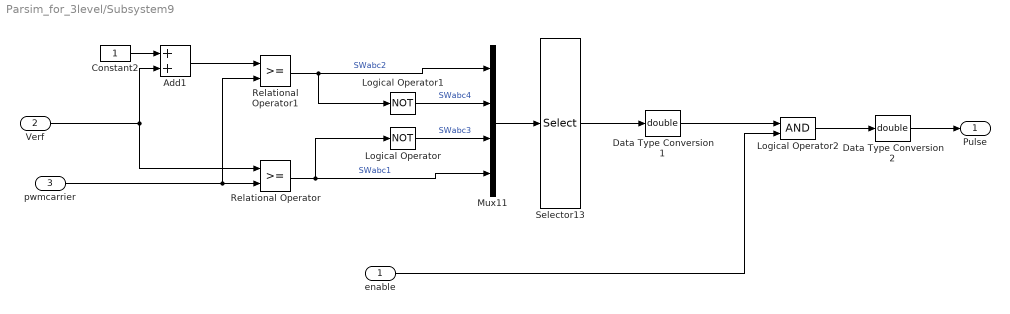
== system Parsim_for_3level/Subsystem9 ==
  enable : Inport
  Verf : Inport  Port=2
  pwmcarrier : Inport  Port=3
  Add1 : Sum
  Constant2 : Constant
  Data Type Conversion1 : DataTypeConversion  OutDataTypeStr=double  SaturateOnIntegerOverflow=off  RndMeth=Floor
  Data Type Conversion2 : DataTypeConversion  OutDataTypeStr=double  SaturateOnIntegerOverflow=off  RndMeth=Floor
  Logical Operator : Logic  Operator=NOT  AllPortsSameDT=off  OutDataTypeStr=boolean
  Logical Operator1 : Logic  Operator=NOT  AllPortsSameDT=off  OutDataTypeStr=boolean
  Logical Operator2 : Logic  AllPortsSameDT=off
  Mux11 : Mux
  Relational Operator : RelationalOperator  OutDataTypeStr=boolean  RndMeth=Simplest  InputSameDT=off
  Relational Operator1 : RelationalOperator  OutDataTypeStr=boolean  RndMeth=Simplest  InputSameDT=off
  Selector13 : Selector  InputPortWidth=12  IndexOptions=Index vector (dialog)  Indices=[10 1 7 4 11 2 8 5 12 3 9 6]  OutputSizes=1
  Pulse : Outport  VectorParamsAs1DForOutWhenUnconnected=off
  wires:
  pwmcarrier/1 -> Relational Operator/2, Relational Operator1/2
  Relational Operator1/1 -> Mux11/1, Logical Operator1/1  "SWabc2"
  Logical Operator/1 -> Mux11/3  "SWabc3"
  Relational Operator/1 -> Logical Operator/1, Mux11/4  "SWabc1"
  Constant2/1 -> Add1/1
  Add1/1 -> Relational Operator1/1
  Verf/1 -> Add1/2, Relational Operator/1
  Selector13/1 -> Data Type Conversion1/1
  Mux11/1 -> Selector13/1
  Logical Operator1/1 -> Mux11/2  "SWabc4"
  Data Type Conversion1/1 -> Logical Operator2/1
  enable/1 -> Logical Operator2/2
  Logical Operator2/1 -> Data Type Conversion2/1
  Data Type Conversion2/1 -> Pulse/1

== system Parsim_for_3level/Rec_VQcontrol1/Vdc ctrl ==
  Vdc : Inport
  Enable : EnablePort  StatesWhenEnabling=reset
  Vdc_ctrler1 : Subsystem
  Pcor_lft : Outport  OutputWhenDisabled=reset  InitialOutput=0  VectorParamsAs1DForOutWhenUnconnected=off
  wires:
  Vdc_ctrler1/1(delP) -> Pcor_lft/1  "Pclft"
  Vdc/1 -> Vdc_ctrler1/1(Vcap)

== system Parsim_for_3level/Rec_VQcontrol1/discrete band pass filter1 ==
  In1 : Inport
  Discrete Transfer Fcn : DiscreteTransferFcn  Numerator=numd  Denominator=dend  InitialStates=inistate  SampleTime=Ts
  Out1 : Outport  VectorParamsAs1DForOutWhenUnconnected=off
  wires:
  Discrete Transfer Fcn/1 -> Out1/1
  In1/1 -> Discrete Transfer Fcn/1

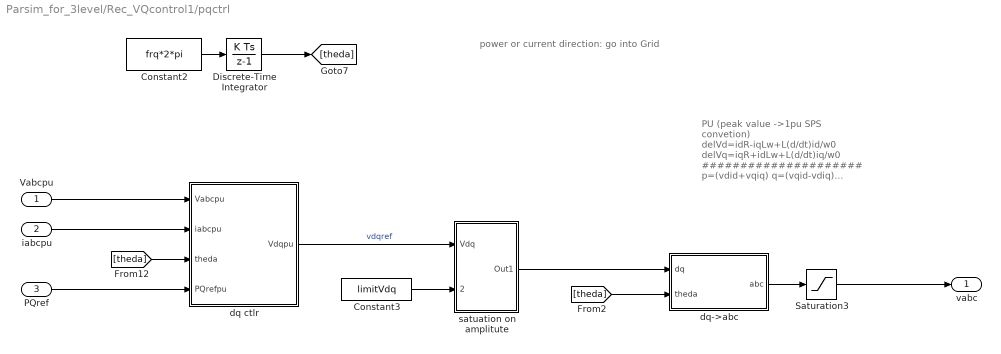
== system Parsim_for_3level/Rec_VQcontrol1/pqctrl ==
  note: PU
      | (peak value ->1pu
      | SPS convetion)
      |
      | delVd=idR-iqLw+L(d/dt)id/w0
      | delVq=iqR+idLw+L(d/dt)iq/w0
      | #####################
      | p=(vdid+vqiq)
      | q=(vqid-vdiq)
      | =>
      | Id=(Vd*P+Vq*Q)/C
      | Iq=(Vq*P-Vd*Q)/C
      | C=Vd^2+Vq^2
  note: power or current direction: go into Grid
  Vabcpu : Inport
  iabcpu : Inport  Port=2
  PQref : Inport  Port=3
  Constant2 : Constant  Value=frq*2*pi
  Constant3 : Constant  Value=limitVdq
  Discrete-Time Integrator : DiscreteIntegrator  SampleTime=Ts  ICPrevOutput=DiscIntNeverNeededParam  ICPrevScaledInput=DiscIntNeverNeededParam
  Saturation3 : Saturate  UpperLimit=Vabc_lim(2)  LowerLimit=Vabc_lim(1)
  dq ctlr : Subsystem
  dq->abc : Subsystem
  "satuation on amplitute " : Subsystem
  vabc : Outport  VectorParamsAs1DForOutWhenUnconnected=off
  wires:
  Saturation3/1 -> vabc/1
  [theda] -> dq->abc/2(theda)
  dq->abc/1(abc) -> Saturation3/1
  Constant3/1 -> "satuation on amplitute "/2(limitVdq)
  "satuation on amplitute "/1(Out1) -> dq->abc/1(dq)
  Constant2/1 -> Discrete-Time Integrator/1
  Discrete-Time Integrator/1 -> [theda]
  [theda] -> dq ctlr/3(theda)
  dq ctlr/1(Vdqpu) -> "satuation on amplitute "/1(Vdq)  "vdqref"
  Vabcpu/1 -> dq ctlr/1(Vabcpu)
  iabcpu/1 -> dq ctlr/2(iabcpu)
  PQref/1 -> dq ctlr/4(PQrefpu)

== system Parsim_for_3level/Rec_VQcontrol3/Vdc ctrl ==
  Vdc : Inport
  Enable : EnablePort  StatesWhenEnabling=reset
  Vdc_ctrler1 : Subsystem
  Pcor_lft : Outport  OutputWhenDisabled=reset  InitialOutput=0  VectorParamsAs1DForOutWhenUnconnected=off
  wires:
  Vdc_ctrler1/1(delP) -> Pcor_lft/1  "Pclft"
  Vdc/1 -> Vdc_ctrler1/1(Vcap)

== system Parsim_for_3level/Rec_VQcontrol3/discrete band pass filter1 ==
  In1 : Inport
  Discrete Transfer Fcn : DiscreteTransferFcn  Numerator=numd  Denominator=dend  InitialStates=inistate  SampleTime=Ts
  Out1 : Outport  VectorParamsAs1DForOutWhenUnconnected=off
  wires:
  Discrete Transfer Fcn/1 -> Out1/1
  In1/1 -> Discrete Transfer Fcn/1

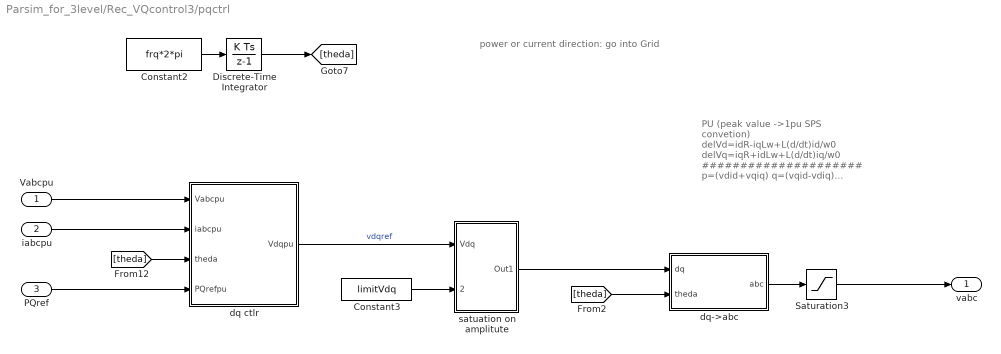
== system Parsim_for_3level/Rec_VQcontrol3/pqctrl ==
  note: PU
      | (peak value ->1pu
      | SPS convetion)
      |
      | delVd=idR-iqLw+L(d/dt)id/w0
      | delVq=iqR+idLw+L(d/dt)iq/w0
      | #####################
      | p=(vdid+vqiq)
      | q=(vqid-vdiq)
      | =>
      | Id=(Vd*P+Vq*Q)/C
      | Iq=(Vq*P-Vd*Q)/C
      | C=Vd^2+Vq^2
  note: power or current direction: go into Grid
  Vabcpu : Inport
  iabcpu : Inport  Port=2
  PQref : Inport  Port=3
  Constant2 : Constant  Value=frq*2*pi
  Constant3 : Constant  Value=limitVdq
  Discrete-Time Integrator : DiscreteIntegrator  SampleTime=Ts  ICPrevOutput=DiscIntNeverNeededParam  ICPrevScaledInput=DiscIntNeverNeededParam
  Saturation3 : Saturate  UpperLimit=Vabc_lim(2)  LowerLimit=Vabc_lim(1)
  dq ctlr : Subsystem
  dq->abc : Subsystem
  "satuation on amplitute " : Subsystem
  vabc : Outport  VectorParamsAs1DForOutWhenUnconnected=off
  wires:
  Saturation3/1 -> vabc/1
  [theda] -> dq->abc/2(theda)
  dq->abc/1(abc) -> Saturation3/1
  Constant3/1 -> "satuation on amplitute "/2(limitVdq)
  "satuation on amplitute "/1(Out1) -> dq->abc/1(dq)
  Constant2/1 -> Discrete-Time Integrator/1
  Discrete-Time Integrator/1 -> [theda]
  [theda] -> dq ctlr/3(theda)
  dq ctlr/1(Vdqpu) -> "satuation on amplitute "/1(Vdq)  "vdqref"
  Vabcpu/1 -> dq ctlr/1(Vabcpu)
  iabcpu/1 -> dq ctlr/2(iabcpu)
  PQref/1 -> dq ctlr/4(PQrefpu)

== system Parsim_for_3level/Rec_VQcontrol1/Vdc ctrl/Vdc_ctrler1 ==
  Vcap : Inport
  Add2 : Sum  Inputs=+-
  PI_d2 : Subsystem  AncestorBlock=|  DialogController=POWERSYS.PowerSysDialog  mask(Discrete PI Controller){Kp=Kvdc(1), Ki=Kvdc(2), Par_Limits=[1 -1]*1, Init=0, Ts=Ts}
      | powerlib_extras/Discrete 
      | Control Blocks/Discrete
      | PI Controller
      mask prompts: Kp "Proportional gain (Kp):"; Ki "Integral gain (Ki):"; Par_Limits "Output limits: [ Upper   Lower ]"; Init "Output initial value:"; Ts "Sample time:"
      mask help: This block implements a discrete PI controller.
      mask init:
      | UpperLimit=Par_Limits(1);
      | LowerLimit=Par_Limits(2);
      | power_initmask();
      mask Help: This block is part of a subset of blocks in the Extras library that does not have documentation associated with it, other than the block mask description.
      mask Display: disp('PI');
  Saturation : Saturate  UpperLimit=0.1  LowerLimit=-0.1
      settings: AttributesFormatString=%<LowerLimit>~%<UpperLimit>
  Vdcpuref : Constant
  Vdctrl : Scope  NumInputPorts=2
  delP : Outport  OutputWhenDisabled=reset  InitialOutput=[0]  VectorParamsAs1DForOutWhenUnconnected=off
  wires:
  PI_d2/1(Out) -> delP/1, Vdctrl/2  "PIVdc"
  Saturation/1 -> PI_d2/1(Error)
  Vdcpuref/1 -> Add2/2
  Vcap/1 -> Add2/1, Vdctrl/1
  Add2/1 -> Saturation/1  "delVdc"

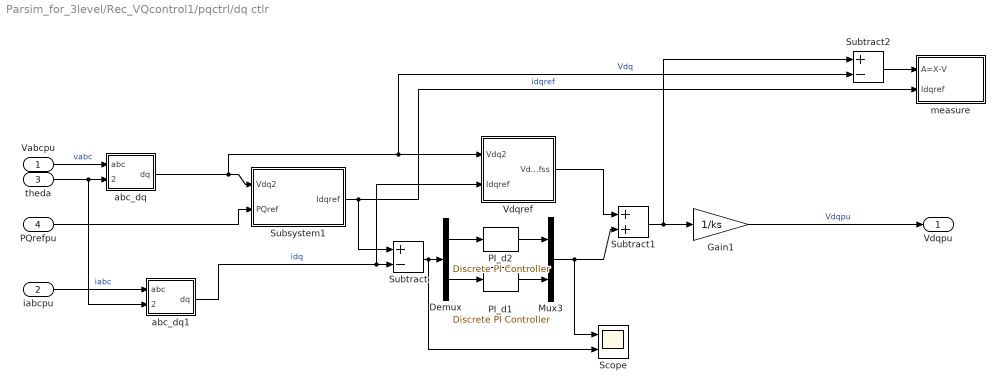
== system Parsim_for_3level/Rec_VQcontrol1/pqctrl/dq ctlr ==
  Vabcpu : Inport
  iabcpu : Inport  Port=2
  theda : Inport  Port=3
  PQrefpu : Inport  Port=4
  Demux : Demux  Outputs=2
  Gain1 : Gain  Gain=1/ks
  Mux3 : Mux  Inputs=2
  PI_d1 : powerlib_extras/Discrete  Control Blocks/Discrete PI Controller  Kp=Kp(1)  Ki=Kp(2)  Par_Limits=[1 -1]*0.15  Init=0  Ts=Ts
  PI_d2 : powerlib_extras/Discrete  Control Blocks/Discrete PI Controller  Kp=Kd(1)  Ki=Kd(2)  Par_Limits=[1 -1]*0.25  Init=0  Ts=Ts
  Scope : Scope  NumInputPorts=2
  Subsystem1 : Subsystem
  Subtract : Sum  Inputs=+-
  Subtract1 : Sum
  Subtract2 : Sum  Inputs=+-
  Vdqref : Subsystem
  abc_dq : Subsystem
  abc_dq1 : Subsystem
  measure : Subsystem
  Vdqpu : Outport  VectorParamsAs1DForOutWhenUnconnected=off
  wires:
  Subtract2/1 -> measure/1(A=X-V)
  Subsystem1/1(Idqref) -> measure/2(Idqref), Subtract/1  "idqref"
  abc_dq/1(dq) -> Subtract2/2, Vdqref/1(Vdq2), Subsystem1/1(Vdq2)  "Vdq"
  abc_dq1/1(dq) -> Vdqref/2(Idqref), Subtract/2  "idq"
  Subtract/1 -> Scope/2, Demux/1
  Demux/1 -> PI_d2/1
  Demux/2 -> PI_d1/1
  Vdqref/1(Vdqrefss) -> Subtract1/1
  PI_d2/1 -> Mux3/1
  PI_d1/1 -> Mux3/2
  Mux3/1 -> Scope/1, Subtract1/2
  Subtract1/1 -> Subtract2/1, Gain1/1
  Vabcpu/1 -> abc_dq/1(abc)  "vabc"
  theda/1 -> abc_dq/2(theta), abc_dq1/2(theta)
  PQrefpu/1 -> Subsystem1/2(PQref)
  iabcpu/1 -> abc_dq1/1(abc)  "iabc"
  Gain1/1 -> Vdqpu/1  "Vdqpu"

== system Parsim_for_3level/Rec_VQcontrol1/pqctrl/dq->abc ==
  note: Va= Vd*sinwt + Vq*cos(wt) + Vo
  note: Vb= Vd*sin(wt-2pi/3) + Vq*cos(wt-2pi/3) + Vo
  note: Vc= Vd*sin(wt+2pi/3) + Vq*cos(wt+2pi/3) + Vo
  dq : Inport
  theda : Inport  Port=2
  Fcn : Fcn  Expr=(u(1)*sin(u(3))+u(2)*cos(u(3)))
  Fcn1 : Fcn  Expr=(u(1)*sin(u(3)-2*pi/3)+u(2)*cos(u(3)-2*pi/3))
  Fcn2 : Fcn  Expr=(u(1)*sin(u(3)+2*pi/3)+u(2)*cos(u(3)+2*pi/3))
  Mux1 : Mux  Inputs=2
  Mux3 : Mux  Inputs=3
  abc : Outport  VectorParamsAs1DForOutWhenUnconnected=off
  wires:
  Fcn2/1 -> Mux3/3
  Fcn1/1 -> Mux3/2
  Fcn/1 -> Mux3/1
  Mux1/1 -> Fcn/1, Fcn2/1, Fcn1/1
  dq/1 -> Mux1/1
  theda/1 -> Mux1/2
  Mux3/1 -> abc/1  "abc"

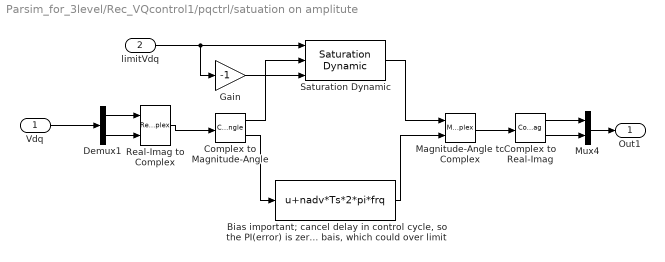
== system Parsim_for_3level/Rec_VQcontrol1/pqctrl/satuation on amplitute  ==
  Vdq : Inport
  limitVdq : Inport  Port=2
  "Bias important; cancel delay in control cycle, so the PI(error) is zero, other wise PI(errer) is bais, which could over limit" : Bias  Bias=nadv*Ts*2*pi*frq  SaturateOnIntegerOverflow=off
  Complex to Magnitude-Angle : ComplexToMagnitudeAngle
  Complex to Real-Imag : ComplexToRealImag
  Demux1 : Demux  Outputs=2
  Gain : Gain  Gain=-1
  Magnitude-Angle to Complex : MagnitudeAngleToComplex
  Mux4 : Mux  Inputs=2
  Real-Imag to Complex : RealImagToComplex
  Saturation Dynamic : simulink/Discontinuities/Saturation Dynamic  OutMin=[]  OutMax=[]  OutDataTypeStr=Inherit: Same as second input  OutDataType=fixdt(1, 16)  OutScaling=2^-10  DoSatur=off
  Out1 : Outport  VectorParamsAs1DForOutWhenUnconnected=off
  wires:
  "Bias important; cancel delay in control cycle, so the PI(error) is zero, other wise PI(errer) is bais, which could over limit"/1 -> Magnitude-Angle to Complex/2
  Gain/1 -> Saturation Dynamic/3
  limitVdq/1 -> Saturation Dynamic/1, Gain/1
  Complex to Magnitude-Angle/1 -> Saturation Dynamic/2
  Saturation Dynamic/1 -> Magnitude-Angle to Complex/1
  Demux1/1 -> Real-Imag to Complex/1
  Demux1/2 -> Real-Imag to Complex/2
  Real-Imag to Complex/1 -> Complex to Magnitude-Angle/1
  Complex to Magnitude-Angle/2 -> "Bias important; cancel delay in control cycle, so the PI(error) is zero, other wise PI(errer) is bais, which could over limit"/1
  Magnitude-Angle to Complex/1 -> Complex to Real-Imag/1
  Complex to Real-Imag/2 -> Mux4/2
  Complex to Real-Imag/1 -> Mux4/1
  Mux4/1 -> Out1/1
  Vdq/1 -> Demux1/1

== system Parsim_for_3level/Rec_VQcontrol3/Vdc ctrl/Vdc_ctrler1 ==
  Vcap : Inport
  Add2 : Sum  Inputs=+-
  PI_d2 : Subsystem  AncestorBlock=|  DialogController=POWERSYS.PowerSysDialog  mask(Discrete PI Controller){Kp=Kvdc(1), Ki=Kvdc(2), Par_Limits=[1 -1]*1, Init=0, Ts=Ts}
      | powerlib_extras/Discrete 
      | Control Blocks/Discrete
      | PI Controller
      mask prompts: Kp "Proportional gain (Kp):"; Ki "Integral gain (Ki):"; Par_Limits "Output limits: [ Upper   Lower ]"; Init "Output initial value:"; Ts "Sample time:"
      mask help: This block implements a discrete PI controller.
      mask init:
      | UpperLimit=Par_Limits(1);
      | LowerLimit=Par_Limits(2);
      | power_initmask();
      mask Help: This block is part of a subset of blocks in the Extras library that does not have documentation associated with it, other than the block mask description.
      mask Display: disp('PI');
  Saturation : Saturate  UpperLimit=0.1  LowerLimit=-0.1
      settings: AttributesFormatString=%<LowerLimit>~%<UpperLimit>
  Vdcpuref : Constant
  Vdctrl : Scope  NumInputPorts=2
  delP : Outport  OutputWhenDisabled=reset  InitialOutput=[0]  VectorParamsAs1DForOutWhenUnconnected=off
  wires:
  PI_d2/1(Out) -> delP/1, Vdctrl/2  "PIVdc"
  Saturation/1 -> PI_d2/1(Error)
  Vdcpuref/1 -> Add2/2
  Vcap/1 -> Add2/1, Vdctrl/1
  Add2/1 -> Saturation/1  "delVdc"

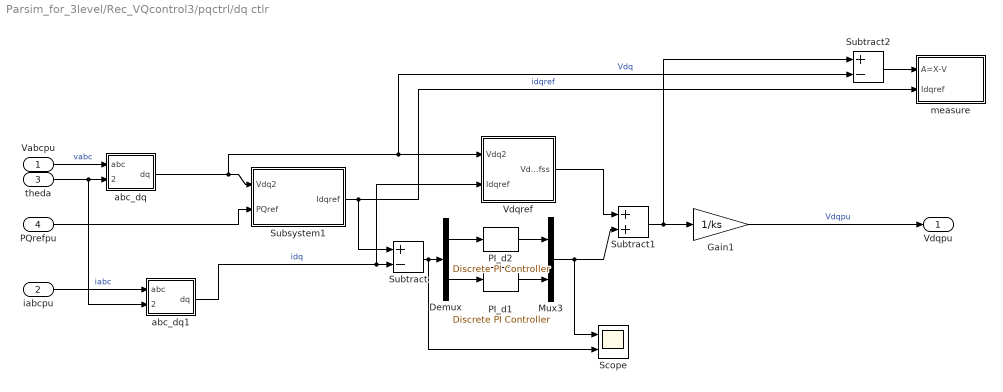
== system Parsim_for_3level/Rec_VQcontrol3/pqctrl/dq ctlr ==
  Vabcpu : Inport
  iabcpu : Inport  Port=2
  theda : Inport  Port=3
  PQrefpu : Inport  Port=4
  Demux : Demux  Outputs=2
  Gain1 : Gain  Gain=1/ks
  Mux3 : Mux  Inputs=2
  PI_d1 : powerlib_extras/Discrete  Control Blocks/Discrete PI Controller  Kp=Kp(1)  Ki=Kp(2)  Par_Limits=[1 -1]*0.15  Init=0  Ts=Ts
  PI_d2 : powerlib_extras/Discrete  Control Blocks/Discrete PI Controller  Kp=Kd(1)  Ki=Kd(2)  Par_Limits=[1 -1]*0.25  Init=0  Ts=Ts
  Scope : Scope  NumInputPorts=2
  Subsystem1 : Subsystem
  Subtract : Sum  Inputs=+-
  Subtract1 : Sum
  Subtract2 : Sum  Inputs=+-
  Vdqref : Subsystem
  abc_dq : Subsystem
  abc_dq1 : Subsystem
  measure : Subsystem
  Vdqpu : Outport  VectorParamsAs1DForOutWhenUnconnected=off
  wires:
  Subtract2/1 -> measure/1(A=X-V)
  Subsystem1/1(Idqref) -> measure/2(Idqref), Subtract/1  "idqref"
  abc_dq/1(dq) -> Subtract2/2, Vdqref/1(Vdq2), Subsystem1/1(Vdq2)  "Vdq"
  abc_dq1/1(dq) -> Vdqref/2(Idqref), Subtract/2  "idq"
  Subtract/1 -> Scope/2, Demux/1
  Demux/1 -> PI_d2/1
  Demux/2 -> PI_d1/1
  Vdqref/1(Vdqrefss) -> Subtract1/1
  PI_d2/1 -> Mux3/1
  PI_d1/1 -> Mux3/2
  Mux3/1 -> Scope/1, Subtract1/2
  Subtract1/1 -> Subtract2/1, Gain1/1
  Vabcpu/1 -> abc_dq/1(abc)  "vabc"
  theda/1 -> abc_dq/2(theta), abc_dq1/2(theta)
  PQrefpu/1 -> Subsystem1/2(PQref)
  iabcpu/1 -> abc_dq1/1(abc)  "iabc"
  Gain1/1 -> Vdqpu/1  "Vdqpu"

== system Parsim_for_3level/Rec_VQcontrol3/pqctrl/dq->abc ==
  note: Va= Vd*sinwt + Vq*cos(wt) + Vo
  note: Vb= Vd*sin(wt-2pi/3) + Vq*cos(wt-2pi/3) + Vo
  note: Vc= Vd*sin(wt+2pi/3) + Vq*cos(wt+2pi/3) + Vo
  dq : Inport
  theda : Inport  Port=2
  Fcn : Fcn  Expr=(u(1)*sin(u(3))+u(2)*cos(u(3)))
  Fcn1 : Fcn  Expr=(u(1)*sin(u(3)-2*pi/3)+u(2)*cos(u(3)-2*pi/3))
  Fcn2 : Fcn  Expr=(u(1)*sin(u(3)+2*pi/3)+u(2)*cos(u(3)+2*pi/3))
  Mux1 : Mux  Inputs=2
  Mux3 : Mux  Inputs=3
  abc : Outport  VectorParamsAs1DForOutWhenUnconnected=off
  wires:
  Fcn2/1 -> Mux3/3
  Fcn1/1 -> Mux3/2
  Fcn/1 -> Mux3/1
  Mux1/1 -> Fcn/1, Fcn2/1, Fcn1/1
  dq/1 -> Mux1/1
  theda/1 -> Mux1/2
  Mux3/1 -> abc/1  "abc"

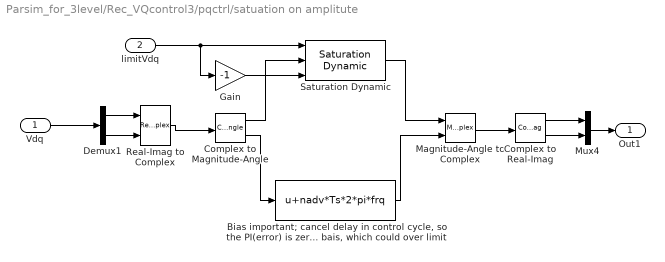
== system Parsim_for_3level/Rec_VQcontrol3/pqctrl/satuation on amplitute  ==
  Vdq : Inport
  limitVdq : Inport  Port=2
  "Bias important; cancel delay in control cycle, so the PI(error) is zero, other wise PI(errer) is bais, which could over limit" : Bias  Bias=nadv*Ts*2*pi*frq  SaturateOnIntegerOverflow=off
  Complex to Magnitude-Angle : ComplexToMagnitudeAngle
  Complex to Real-Imag : ComplexToRealImag
  Demux1 : Demux  Outputs=2
  Gain : Gain  Gain=-1
  Magnitude-Angle to Complex : MagnitudeAngleToComplex
  Mux4 : Mux  Inputs=2
  Real-Imag to Complex : RealImagToComplex
  Saturation Dynamic : simulink/Discontinuities/Saturation Dynamic  OutMin=[]  OutMax=[]  OutDataTypeStr=Inherit: Same as second input  OutDataType=fixdt(1, 16)  OutScaling=2^-10  DoSatur=off
  Out1 : Outport  VectorParamsAs1DForOutWhenUnconnected=off
  wires:
  "Bias important; cancel delay in control cycle, so the PI(error) is zero, other wise PI(errer) is bais, which could over limit"/1 -> Magnitude-Angle to Complex/2
  Gain/1 -> Saturation Dynamic/3
  limitVdq/1 -> Saturation Dynamic/1, Gain/1
  Complex to Magnitude-Angle/1 -> Saturation Dynamic/2
  Saturation Dynamic/1 -> Magnitude-Angle to Complex/1
  Demux1/1 -> Real-Imag to Complex/1
  Demux1/2 -> Real-Imag to Complex/2
  Real-Imag to Complex/1 -> Complex to Magnitude-Angle/1
  Complex to Magnitude-Angle/2 -> "Bias important; cancel delay in control cycle, so the PI(error) is zero, other wise PI(errer) is bais, which could over limit"/1
  Magnitude-Angle to Complex/1 -> Complex to Real-Imag/1
  Complex to Real-Imag/2 -> Mux4/2
  Complex to Real-Imag/1 -> Mux4/1
  Mux4/1 -> Out1/1
  Vdq/1 -> Demux1/1

== system Parsim_for_3level/Rec_VQcontrol1/Vdc ctrl/Vdc_ctrler1/PI_d2 ==
  note: Discrete PID Controller
  note: Pierre Giroux, Gilbert Sybille
      | Power System Simulation Laboratory
      | IREQ, Hydro-Quebc
  Error : Inport  SampleTime=Ts
  Discrete-Time Integrator : DiscreteIntegrator  InitialCondition=Init  SampleTime=Ts  LimitOutput=on  UpperSaturationLimit=UpperLimit  LowerSaturationLimit=LowerLimit  ICPrevOutput=DiscIntNeverNeededParam  ICPrevScaledInput=DiscIntNeverNeededParam
  Kp4 : Gain  Gain=Kp  SaturateOnIntegerOverflow=on  SampleTime=Ts  OutDataTypeStr=Inherit: Same as input  ParamDataTypeStr=Inherit: Same as input
  Kp5 : Gain  Gain=Ki  SaturateOnIntegerOverflow=on  SampleTime=Ts  OutDataTypeStr=Inherit: Same as input  ParamDataTypeStr=Inherit: Same as input
  Saturation2 : Saturate  UpperLimit=UpperLimit  LowerLimit=LowerLimit  SampleTime=Ts
  Sum6 : Sum  InputSameDT=on  SaturateOnIntegerOverflow=on  SampleTime=Ts  OutDataTypeStr=Inherit: Same as first input
  Zero-Order Hold : ZeroOrderHold  SampleTime=Ts
  Out : Outport  SampleTime=Ts  InitialOutput=0  VectorParamsAs1DForOutWhenUnconnected=off
  wires:
  Zero-Order Hold/1 -> Sum6/1  "prop"
  Saturation2/1 -> Out/1
  Discrete-Time Integrator/1 -> Sum6/2  "int"
  Kp4/1 -> Zero-Order Hold/1
  Kp5/1 -> Discrete-Time Integrator/1
  Sum6/1 -> Saturation2/1
  Error/1 -> Kp5/1, Kp4/1

== system Parsim_for_3level/Rec_VQcontrol1/pqctrl/dq ctlr/Subsystem1 ==
  Vdq2 : Inport
  PQref : Inport  Port=2
  Fcn7 : Fcn  Expr=(u[1] *u[4]+u[2]*u[5])/u[3]
  Fcn8 : Fcn  Expr=(u[2] *u[4]-u[1]*u[5])/u[3]
  Fcn9 : Fcn  Expr=(u[1] ^2+u[2]^2)
  Mux3 : Mux  Inputs=[2 1 2]
  Mux4 : Mux  Inputs=2
  Saturation : Saturate  UpperLimit=inf  LowerLimit=0.01
  Saturation1 : Saturate  UpperLimit=1.5  LowerLimit=-1.5
  Idqref : Outport  VectorParamsAs1DForOutWhenUnconnected=off
  wires:
  Saturation1/1 -> Idqref/1
  Vdq2/1 -> Fcn9/1, Mux3/1
  Mux3/1 -> Fcn8/1, Fcn7/1
  Fcn9/1 -> Saturation/1
  Fcn7/1 -> Mux4/1
  Fcn8/1 -> Mux4/2
  Mux4/1 -> Saturation1/1  "Idqref"
  PQref/1 -> Mux3/3
  Saturation/1 -> Mux3/2

== system Parsim_for_3level/Rec_VQcontrol1/pqctrl/dq ctlr/Vdqref ==
  Vdq2 : Inport
  Idqref : Inport  Port=2
  Display : Display
      settings: Decimation=50
  Fcn7 : Fcn  Expr=(u[2] +u[4]*u[5]+u[3]*u[6])
  Fcn8 : Fcn  Expr=(u[1] +u[3]*u[5]-u[4]*u[6])
  Lxpu : Constant  Value=Lxpu
  Mux3 : Mux
  Mux4 : Mux  Inputs=2
  Rxpu : Constant  Value=Rxpu
  Vdqrefss : Outport  VectorParamsAs1DForOutWhenUnconnected=off
  wires:
  Lxpu/1 -> Mux3/4
  Rxpu/1 -> Mux3/3
  Mux3/1 -> Display/1, Fcn8/1, Fcn7/1
  Fcn8/1 -> Mux4/1  "Vdref"
  Fcn7/1 -> Mux4/2  "Vqref"
  Vdq2/1 -> Mux3/1
  Idqref/1 -> Mux3/2
  Mux4/1 -> Vdqrefss/1

== system Parsim_for_3level/Rec_VQcontrol1/pqctrl/dq ctlr/abc_dq ==
  abc : Inport
  theta : Inport  Port=2
  Mux2 : Mux  Inputs=2
  Selector3 : Selector  InputPortWidth=3  IndexOptions=Index vector (dialog)  Indices=[1 2]  OutputSizes=1
  Trigonometric Function2 : Trigonometry
  Trigonometric Function3 : Trigonometry  Operator=cos
  abc/dq1 : powerlib_extras/Measurements/abc_to_dq0 Transformation
  dq : Outport  VectorParamsAs1DForOutWhenUnconnected=off
  wires:
  abc/1 -> abc/dq1/1
  Selector3/1 -> dq/1
  abc/dq1/1 -> Selector3/1
  Mux2/1 -> abc/dq1/2
  theta/1 -> Trigonometric Function3/1, Trigonometric Function2/1
  Trigonometric Function2/1 -> Mux2/1
  Trigonometric Function3/1 -> Mux2/2

== system Parsim_for_3level/Rec_VQcontrol1/pqctrl/dq ctlr/abc_dq1 ==
  abc : Inport
  theta : Inport  Port=2
  Mux2 : Mux  Inputs=2
  Selector3 : Selector  InputPortWidth=3  IndexOptions=Index vector (dialog)  Indices=[1 2]  OutputSizes=1
  Trigonometric Function2 : Trigonometry
  Trigonometric Function3 : Trigonometry  Operator=cos
  abc/dq1 : powerlib_extras/Measurements/abc_to_dq0 Transformation
  dq : Outport  VectorParamsAs1DForOutWhenUnconnected=off
  wires:
  Trigonometric Function3/1 -> Mux2/2
  Trigonometric Function2/1 -> Mux2/1
  theta/1 -> Trigonometric Function2/1, Trigonometric Function3/1
  Mux2/1 -> abc/dq1/2
  abc/dq1/1 -> Selector3/1
  Selector3/1 -> dq/1
  abc/1 -> abc/dq1/1
